simulink library "monroe_library"  (R2012b)
settings: Solver=ode45  StartTime=0.0  StopTime=10.0  RelTol=1e-3
values from neighbouring files (symbols this model uses):
  input_bit_width = ', num2str(input_bit_width))    [fft_direct_draw.m]
undefined symbols (not defined in the file or in its folder): gcbh, xlBlockLoadCallback
libraries: xbsIndex_r4 x1880, monroe_library x159, casper_library x13, xps_library x1
(part 39 of 43)

== system monroe_library/FFT_direct/direct_coeff_gen/coeff_gen_stage_3_group_2 ==
  sync : Inport
  Concat : xbsIndex_r4/Concat  num_inputs=2  dbl_ovrd=off  block_type=concat
  Concat1 : xbsIndex_r4/Concat  num_inputs=2  dbl_ovrd=off  block_type=concat
  Concat2 : xbsIndex_r4/Concat  num_inputs=2  dbl_ovrd=off  block_type=concat
  Constant : xbsIndex_r4/Constant  arith_type=Boolean  const=0  n_bits=16  bin_pt=14  explicit_period=on  period=1  equ=P=C  opselect=C  inp2=PCIN>>17  opr=+  inp1=P  carry=CIN  dbl_ovrd=off  block_type=constant
  Constant1 : xbsIndex_r4/Constant  arith_type=Boolean  const=1  n_bits=16  bin_pt=14  explicit_period=on  period=1  equ=P=C  opselect=C  inp2=PCIN>>17  opr=+  inp1=P  carry=CIN  dbl_ovrd=off  block_type=constant
  Constant3 : xbsIndex_r4/Constant  arith_type=Signed (2's comp)  const=0  n_bits=18  bin_pt=17  explicit_period=on  period=1  equ=P=C  opselect=C  inp2=PCIN>>17  opr=+  inp1=P  carry=CIN  dbl_ovrd=off  block_type=constant
  Constant4 : xbsIndex_r4/Constant  arith_type=Boolean  const=0  n_bits=16  bin_pt=14  explicit_period=on  period=1  equ=P=C  opselect=C  inp2=PCIN>>17  opr=+  inp1=P  carry=CIN  dbl_ovrd=off  block_type=constant
  Counter : xbsIndex_r4/Counter  cnt_type=Free Running  cnt_to=Inf  operation=Up  start_count=3  cnt_by_val=1  arith_type=Unsigned  n_bits=6  bin_pt=0  load_pin=off  rst=on  en=off  explicit_period=on  period=1  dbl_ovrd=off  use_behavioral_HDL=off  implementation=Fabric  block_type=counter
  Delay : xbsIndex_r4/Delay  en=off  latency=1  dbl_ovrd=off  reg_retiming=off  block_type=delay
  Dual Port RAM4 : xbsIndex_r4/Dual Port RAM  depth=128  initVector=[-1 -0.999924701839145 -0.999698818696204 -0.99932238458835 -0.998795456205172 -0.998118112900149 -0.99729045667869 -0.996312612182778 -0.995184726672197 -0.993906970002356 -0.99247953459871 -0.99090263542778 -0.989176509964781 -0.987301418157858 -0.985277642388941 -0.983105487431216 -0.98078528040323 -0.978317370719628 -0.975702130038529 -0.97293995220556 -0.970031253194544 -0.966976471044852 -0.96377606579544 -0.960430519415566 -0.956940335732209 -0.953306040354194 -0.949528180593037 -0.945607325380521 -0.941544065183021 -0.937339011912575 -0.932992798834739 -0.928506080473216 -0.923879532511287 -0.919113851690058 -0.914209755703531 -0.909167983090522 -0.903989293123443 -0.898674465693954 -0.893224301195515 -0.887639620402854 -0.881921264348355 -0.876070094195407 -0.870086991108711 -0.863972856121587 -0.857728610000272 -0.851355193105265 -0.844853565249707 -0.838224705554838 -0.831469612302545 -0.824589302785025 -0.817584813151584 -0.810457198252595 -0.803207531480645 -0.795836904608884 -0.788346427626606 -0.780737228572095 -0.773010453362737 -0.765167265622459 -0.757208846506485 -0.749136394523459 -0.740951125354959 -0.732654271672413 -0.724247082951467 -0.715730825283819 6.12323399573677e-017 -0.0122715382857198 -0.0245412285229121 -0.0368072229413589 -0.049067674327418 -0.0613207363022085 -0.0735645635996673 -0.0857973123444398 -0.0980171403295606 -0.110222207293883 -0.122410675199216 -0.134580708507126 -0.146730474455362 -0.158858143333861 -0.170961888760301 -0.183039887955141 -0.195090322016128 -0.207111376192218 -0.21910124015687 -0.231058108280671 -0.242980179903264 -0.254865659604515 -0.266712757474898 -0.278519689385053 -0.290284677254462 -0.302005949319228 -0.313681740398891 -0.325310292162263 -0.33688985339222 -0.348418680249434 -0.359895036534988 -0.371317193951837 -0.38268343236509 -0.393992040061048 -0.40524131400499 -0.416429560097637 -0.427555093430282 -0.438616238538527 -0.449611329654607 -0.46053871095824 -0.471396736825998 -0.482183772079123 -0.492898192229784 -0.503538383725717 -0.514102744193222 -0.524589682678469 -0.534997619887097 -0.545324988422046 -0.555570233019602 -0.565731810783613 -0.575808191417845 -0.585797857456439 -0.595699304492433 -0.605511041404325 -0.615231590580627 -0.624859488142386 -0.634393284163645 -0.643831542889791 -0.653172842953777 -0.662415777590172 -0.671558954847018 -0.680600997795453 -0.689540544737067 -0.698376249408973]  distributed_mem=Block RAM  init_a=0  init_b=0  rst_a=off  rst_b=off  en_a=off  en_b=off  latency=2  write_mode_A=No Read On Write  write_mode_B=No Read On Write  dbl_ovrd=off  optimize=Area  use_rpm=on  block_type=dpram
  Reinterpret : xbsIndex_r4/Reinterpret  force_arith_type=on  arith_type=Unsigned  force_bin_pt=on  bin_pt=0  block_type=reinterpret
      settings: infoedit="Changes signal type without altering the binary representation.   You can changed the signal between signed and unsigned, and relocate the binary point.<br><br>Hardware notes: In hardware this block costs nothing.<br><br>Example:  Suppose the input is 6 bits wide, signed, with 2 fractional bits, and the output is forced to unsigned with 0 fractional bits.  Then an input of -2.0 (1110.00 in binary 2's complement) becomes an output of 56 (111000 in binary)."
  Reinterpret1 : xbsIndex_r4/Reinterpret  force_arith_type=on  arith_type=Unsigned  force_bin_pt=on  bin_pt=0  block_type=reinterpret
      settings: infoedit="Changes signal type without altering the binary representation.   You can changed the signal between signed and unsigned, and relocate the binary point.<br><br>Hardware notes: In hardware this block costs nothing.<br><br>Example:  Suppose the input is 6 bits wide, signed, with 2 fractional bits, and the output is forced to unsigned with 0 fractional bits.  Then an input of -2.0 (1110.00 in binary 2's complement) becomes an output of 56 (111000 in binary)."
  count_slice : xbsIndex_r4/Slice  nbits=6  boolean_output=off  mode=Upper Bit Location + Width  bit1=0  base1=MSB of Input  bit0=0  base0=MSB of Input  dbl_ovrd=off  block_type=slice
  coeff : Outport
  wires:
  count_slice/1 -> Concat1/2, Concat/2
  Constant3/1 -> Dual Port RAM4/5, Dual Port RAM4/2
  Constant/1 -> Dual Port RAM4/6, Dual Port RAM4/3
  Reinterpret1/1 -> Concat2/2
  Dual Port RAM4/2 -> Reinterpret1/1  "xlsub2_Dual_Port_RAM4_out2"
  Reinterpret/1 -> Concat2/1
  Dual Port RAM4/1 -> Reinterpret/1  "xlsub2_Dual_Port_RAM4_out1"
  Concat1/1 -> Dual Port RAM4/4
  Concat/1 -> Dual Port RAM4/1
  Delay/1 -> coeff/1
  Concat2/1 -> Delay/1
  Constant4/1 -> Concat1/1
  Constant1/1 -> Concat/1
  Counter/1 -> count_slice/1
  sync/1 -> Counter/1

== system monroe_library/FFT_direct/direct_coeff_gen/coeff_gen_stage_3_group_3 ==
  sync : Inport
  Concat : xbsIndex_r4/Concat  num_inputs=2  dbl_ovrd=off  block_type=concat
  Concat1 : xbsIndex_r4/Concat  num_inputs=2  dbl_ovrd=off  block_type=concat
  Concat2 : xbsIndex_r4/Concat  num_inputs=2  dbl_ovrd=off  block_type=concat
  Constant : xbsIndex_r4/Constant  arith_type=Boolean  const=0  n_bits=16  bin_pt=14  explicit_period=on  period=1  equ=P=C  opselect=C  inp2=PCIN>>17  opr=+  inp1=P  carry=CIN  dbl_ovrd=off  block_type=constant
  Constant1 : xbsIndex_r4/Constant  arith_type=Boolean  const=1  n_bits=16  bin_pt=14  explicit_period=on  period=1  equ=P=C  opselect=C  inp2=PCIN>>17  opr=+  inp1=P  carry=CIN  dbl_ovrd=off  block_type=constant
  Constant3 : xbsIndex_r4/Constant  arith_type=Signed (2's comp)  const=0  n_bits=18  bin_pt=17  explicit_period=on  period=1  equ=P=C  opselect=C  inp2=PCIN>>17  opr=+  inp1=P  carry=CIN  dbl_ovrd=off  block_type=constant
  Constant4 : xbsIndex_r4/Constant  arith_type=Boolean  const=0  n_bits=16  bin_pt=14  explicit_period=on  period=1  equ=P=C  opselect=C  inp2=PCIN>>17  opr=+  inp1=P  carry=CIN  dbl_ovrd=off  block_type=constant
  Counter : xbsIndex_r4/Counter  cnt_type=Free Running  cnt_to=Inf  operation=Up  start_count=3  cnt_by_val=1  arith_type=Unsigned  n_bits=6  bin_pt=0  load_pin=off  rst=on  en=off  explicit_period=on  period=1  dbl_ovrd=off  use_behavioral_HDL=off  implementation=Fabric  block_type=counter
  Delay : xbsIndex_r4/Delay  en=off  latency=1  dbl_ovrd=off  reg_retiming=off  block_type=delay
  Dual Port RAM4 : xbsIndex_r4/Dual Port RAM  depth=128  initVector=[-0.707106781186547 -0.715730825283819 -0.724247082951467 -0.732654271672413 -0.740951125354959 -0.749136394523459 -0.757208846506485 -0.765167265622459 -0.773010453362737 -0.780737228572094 -0.788346427626606 -0.795836904608884 -0.803207531480645 -0.810457198252595 -0.817584813151584 -0.824589302785025 -0.831469612302545 -0.838224705554838 -0.844853565249707 -0.851355193105265 -0.857728610000272 -0.863972856121587 -0.870086991108711 -0.876070094195407 -0.881921264348355 -0.887639620402854 -0.893224301195515 -0.898674465693954 -0.903989293123443 -0.909167983090522 -0.914209755703531 -0.919113851690058 -0.923879532511287 -0.928506080473216 -0.932992798834739 -0.937339011912575 -0.941544065183021 -0.945607325380521 -0.949528180593037 -0.953306040354194 -0.956940335732209 -0.960430519415566 -0.96377606579544 -0.966976471044852 -0.970031253194544 -0.97293995220556 -0.975702130038529 -0.978317370719628 -0.98078528040323 -0.983105487431216 -0.985277642388941 -0.987301418157858 -0.989176509964781 -0.99090263542778 -0.99247953459871 -0.993906970002356 -0.995184726672197 -0.996312612182778 -0.99729045667869 -0.998118112900149 -0.998795456205172 -0.99932238458835 -0.999698818696204 -0.999924701839145 0.707106781186548 0.698376249408973 0.689540544737067 0.680600997795453 0.671558954847018 0.662415777590172 0.653172842953777 0.643831542889792 0.634393284163645 0.624859488142386 0.615231590580627 0.605511041404326 0.595699304492433 0.585797857456439 0.575808191417845 0.565731810783613 0.555570233019602 0.545324988422046 0.534997619887097 0.524589682678469 0.514102744193222 0.503538383725718 0.492898192229784 0.482183772079123 0.471396736825998 0.46053871095824 0.449611329654607 0.438616238538528 0.427555093430282 0.416429560097637 0.40524131400499 0.393992040061048 0.38268343236509 0.371317193951838 0.359895036534988 0.348418680249435 0.33688985339222 0.325310292162263 0.313681740398892 0.302005949319228 0.290284677254462 0.278519689385053 0.266712757474898 0.254865659604515 0.242980179903264 0.231058108280671 0.21910124015687 0.207111376192219 0.195090322016128 0.183039887955141 0.170961888760301 0.158858143333861 0.146730474455362 0.134580708507126 0.122410675199216 0.110222207293883 0.0980171403295608 0.0857973123444399 0.0735645635996675 0.0613207363022086 0.0490676743274181 0.036807222941359 0.0245412285229123 0.0122715382857199]  distributed_mem=Block RAM  init_a=0  init_b=0  rst_a=off  rst_b=off  en_a=off  en_b=off  latency=2  write_mode_A=No Read On Write  write_mode_B=No Read On Write  dbl_ovrd=off  optimize=Area  use_rpm=on  block_type=dpram
  Reinterpret : xbsIndex_r4/Reinterpret  force_arith_type=on  arith_type=Unsigned  force_bin_pt=on  bin_pt=0  block_type=reinterpret
      settings: infoedit="Changes signal type without altering the binary representation.   You can changed the signal between signed and unsigned, and relocate the binary point.<br><br>Hardware notes: In hardware this block costs nothing.<br><br>Example:  Suppose the input is 6 bits wide, signed, with 2 fractional bits, and the output is forced to unsigned with 0 fractional bits.  Then an input of -2.0 (1110.00 in binary 2's complement) becomes an output of 56 (111000 in binary)."
  Reinterpret1 : xbsIndex_r4/Reinterpret  force_arith_type=on  arith_type=Unsigned  force_bin_pt=on  bin_pt=0  block_type=reinterpret
      settings: infoedit="Changes signal type without altering the binary representation.   You can changed the signal between signed and unsigned, and relocate the binary point.<br><br>Hardware notes: In hardware this block costs nothing.<br><br>Example:  Suppose the input is 6 bits wide, signed, with 2 fractional bits, and the output is forced to unsigned with 0 fractional bits.  Then an input of -2.0 (1110.00 in binary 2's complement) becomes an output of 56 (111000 in binary)."
  count_slice : xbsIndex_r4/Slice  nbits=6  boolean_output=off  mode=Upper Bit Location + Width  bit1=0  base1=MSB of Input  bit0=0  base0=MSB of Input  dbl_ovrd=off  block_type=slice
  coeff : Outport
  wires:
  count_slice/1 -> Concat1/2, Concat/2
  Constant3/1 -> Dual Port RAM4/5, Dual Port RAM4/2
  Constant/1 -> Dual Port RAM4/6, Dual Port RAM4/3
  Reinterpret1/1 -> Concat2/2
  Dual Port RAM4/2 -> Reinterpret1/1  "xlsub2_Dual_Port_RAM4_out2"
  Reinterpret/1 -> Concat2/1
  Dual Port RAM4/1 -> Reinterpret/1  "xlsub2_Dual_Port_RAM4_out1"
  Concat1/1 -> Dual Port RAM4/4
  Concat/1 -> Dual Port RAM4/1
  Delay/1 -> coeff/1
  Concat2/1 -> Delay/1
  Constant4/1 -> Concat1/1
  Constant1/1 -> Concat/1
  Counter/1 -> count_slice/1
  sync/1 -> Counter/1

== system monroe_library/FFT_direct/direct_coeff_gen/coeff_gen_stage_3_group_4 ==
  sync : Inport
  Concat : xbsIndex_r4/Concat  num_inputs=2  dbl_ovrd=off  block_type=concat
  Concat1 : xbsIndex_r4/Concat  num_inputs=2  dbl_ovrd=off  block_type=concat
  Concat2 : xbsIndex_r4/Concat  num_inputs=2  dbl_ovrd=off  block_type=concat
  Constant : xbsIndex_r4/Constant  arith_type=Boolean  const=0  n_bits=16  bin_pt=14  explicit_period=on  period=1  equ=P=C  opselect=C  inp2=PCIN>>17  opr=+  inp1=P  carry=CIN  dbl_ovrd=off  block_type=constant
  Constant1 : xbsIndex_r4/Constant  arith_type=Boolean  const=1  n_bits=16  bin_pt=14  explicit_period=on  period=1  equ=P=C  opselect=C  inp2=PCIN>>17  opr=+  inp1=P  carry=CIN  dbl_ovrd=off  block_type=constant
  Constant3 : xbsIndex_r4/Constant  arith_type=Signed (2's comp)  const=0  n_bits=18  bin_pt=17  explicit_period=on  period=1  equ=P=C  opselect=C  inp2=PCIN>>17  opr=+  inp1=P  carry=CIN  dbl_ovrd=off  block_type=constant
  Constant4 : xbsIndex_r4/Constant  arith_type=Boolean  const=0  n_bits=16  bin_pt=14  explicit_period=on  period=1  equ=P=C  opselect=C  inp2=PCIN>>17  opr=+  inp1=P  carry=CIN  dbl_ovrd=off  block_type=constant
  Counter : xbsIndex_r4/Counter  cnt_type=Free Running  cnt_to=Inf  operation=Up  start_count=3  cnt_by_val=1  arith_type=Unsigned  n_bits=6  bin_pt=0  load_pin=off  rst=on  en=off  explicit_period=on  period=1  dbl_ovrd=off  use_behavioral_HDL=off  implementation=Fabric  block_type=counter
  Delay : xbsIndex_r4/Delay  en=off  latency=1  dbl_ovrd=off  reg_retiming=off  block_type=delay
  Dual Port RAM4 : xbsIndex_r4/Dual Port RAM  depth=128  initVector=[-0.707106781186548 -0.698376249408973 -0.689540544737067 -0.680600997795453 -0.671558954847019 -0.662415777590172 -0.653172842953777 -0.643831542889791 -0.634393284163645 -0.624859488142386 -0.615231590580627 -0.605511041404326 -0.595699304492433 -0.585797857456439 -0.575808191417845 -0.565731810783613 -0.555570233019602 -0.545324988422046 -0.534997619887097 -0.524589682678469 -0.514102744193222 -0.503538383725718 -0.492898192229784 -0.482183772079123 -0.471396736825998 -0.46053871095824 -0.449611329654607 -0.438616238538528 -0.427555093430282 -0.416429560097637 -0.40524131400499 -0.393992040061048 -0.38268343236509 -0.371317193951838 -0.359895036534988 -0.348418680249435 -0.33688985339222 -0.325310292162263 -0.313681740398891 -0.302005949319228 -0.290284677254462 -0.278519689385053 -0.266712757474898 -0.254865659604515 -0.242980179903264 -0.231058108280671 -0.21910124015687 -0.207111376192219 -0.195090322016129 -0.183039887955141 -0.170961888760301 -0.158858143333861 -0.146730474455362 -0.134580708507126 -0.122410675199216 -0.110222207293883 -0.0980171403295608 -0.0857973123444402 -0.0735645635996677 -0.0613207363022085 -0.049067674327418 -0.0368072229413588 -0.0245412285229123 -0.01227153828572 -0.707106781186547 -0.715730825283819 -0.724247082951467 -0.732654271672413 -0.740951125354959 -0.749136394523459 -0.757208846506485 -0.765167265622459 -0.773010453362737 -0.780737228572094 -0.788346427626606 -0.795836904608883 -0.803207531480645 -0.810457198252595 -0.817584813151584 -0.824589302785025 -0.831469612302545 -0.838224705554838 -0.844853565249707 -0.851355193105265 -0.857728610000272 -0.863972856121587 -0.870086991108711 -0.876070094195406 -0.881921264348355 -0.887639620402854 -0.893224301195515 -0.898674465693954 -0.903989293123443 -0.909167983090522 -0.914209755703531 -0.919113851690058 -0.923879532511287 -0.928506080473215 -0.932992798834739 -0.937339011912575 -0.941544065183021 -0.945607325380521 -0.949528180593037 -0.953306040354194 -0.956940335732209 -0.960430519415566 -0.96377606579544 -0.966976471044852 -0.970031253194544 -0.97293995220556 -0.975702130038528 -0.978317370719628 -0.98078528040323 -0.983105487431216 -0.985277642388941 -0.987301418157858 -0.989176509964781 -0.99090263542778 -0.99247953459871 -0.993906970002356 -0.995184726672197 -0.996312612182778 -0.99729045667869 -0.998118112900149 -0.998795456205172 -0.99932238458835 -0.999698818696204 -0.999924701839145]  distributed_mem=Block RAM  init_a=0  init_b=0  rst_a=off  rst_b=off  en_a=off  en_b=off  latency=2  write_mode_A=No Read On Write  write_mode_B=No Read On Write  dbl_ovrd=off  optimize=Area  use_rpm=on  block_type=dpram
  Reinterpret : xbsIndex_r4/Reinterpret  force_arith_type=on  arith_type=Unsigned  force_bin_pt=on  bin_pt=0  block_type=reinterpret
      settings: infoedit="Changes signal type without altering the binary representation.   You can changed the signal between signed and unsigned, and relocate the binary point.<br><br>Hardware notes: In hardware this block costs nothing.<br><br>Example:  Suppose the input is 6 bits wide, signed, with 2 fractional bits, and the output is forced to unsigned with 0 fractional bits.  Then an input of -2.0 (1110.00 in binary 2's complement) becomes an output of 56 (111000 in binary)."
  Reinterpret1 : xbsIndex_r4/Reinterpret  force_arith_type=on  arith_type=Unsigned  force_bin_pt=on  bin_pt=0  block_type=reinterpret
      settings: infoedit="Changes signal type without altering the binary representation.   You can changed the signal between signed and unsigned, and relocate the binary point.<br><br>Hardware notes: In hardware this block costs nothing.<br><br>Example:  Suppose the input is 6 bits wide, signed, with 2 fractional bits, and the output is forced to unsigned with 0 fractional bits.  Then an input of -2.0 (1110.00 in binary 2's complement) becomes an output of 56 (111000 in binary)."
  count_slice : xbsIndex_r4/Slice  nbits=6  boolean_output=off  mode=Upper Bit Location + Width  bit1=0  base1=MSB of Input  bit0=0  base0=MSB of Input  dbl_ovrd=off  block_type=slice
  coeff : Outport
  wires:
  count_slice/1 -> Concat1/2, Concat/2
  Constant3/1 -> Dual Port RAM4/5, Dual Port RAM4/2
  Constant/1 -> Dual Port RAM4/6, Dual Port RAM4/3
  Reinterpret1/1 -> Concat2/2
  Dual Port RAM4/2 -> Reinterpret1/1  "xlsub2_Dual_Port_RAM4_out2"
  Reinterpret/1 -> Concat2/1
  Dual Port RAM4/1 -> Reinterpret/1  "xlsub2_Dual_Port_RAM4_out1"
  Concat1/1 -> Dual Port RAM4/4
  Concat/1 -> Dual Port RAM4/1
  Delay/1 -> coeff/1
  Concat2/1 -> Delay/1
  Constant4/1 -> Concat1/1
  Constant1/1 -> Concat/1
  Counter/1 -> count_slice/1
  sync/1 -> Counter/1

== system monroe_library/FFT_direct/stage_1/uncram_coeff ==
  in : Inport
  signal1 : xbsIndex_r4/Slice  nbits=36  boolean_output=off  mode=Upper Bit Location + Width  bit1=-0  base1=MSB of Input  bit0=-0  base0=MSB of Input  dbl_ovrd=off  block_type=slice
  signal2 : xbsIndex_r4/Slice  nbits=36  boolean_output=off  mode=Upper Bit Location + Width  bit1=-36  base1=MSB of Input  bit0=-36  base0=MSB of Input  dbl_ovrd=off  block_type=slice
  signal3 : xbsIndex_r4/Slice  nbits=36  boolean_output=off  mode=Upper Bit Location + Width  bit1=-72  base1=MSB of Input  bit0=-72  base0=MSB of Input  dbl_ovrd=off  block_type=slice
  signal4 : xbsIndex_r4/Slice  nbits=36  boolean_output=off  mode=Upper Bit Location + Width  bit1=-108  base1=MSB of Input  bit0=-108  base0=MSB of Input  dbl_ovrd=off  block_type=slice
  out0 : Outport
  out1 : Outport  Port=2
  out2 : Outport  Port=3
  out3 : Outport  Port=4
  wires:
  in/1 -> signal4/1, signal3/1, signal2/1, signal1/1
  signal4/1 -> out3/1
  signal3/1 -> out2/1
  signal2/1 -> out1/1
  signal1/1 -> out0/1

== system monroe_library/FFT_direct/stage_2/uncram_coeff ==
  in : Inport
  signal1 : xbsIndex_r4/Slice  nbits=36  boolean_output=off  mode=Upper Bit Location + Width  bit1=-0  base1=MSB of Input  bit0=-0  base0=MSB of Input  dbl_ovrd=off  block_type=slice
  signal2 : xbsIndex_r4/Slice  nbits=36  boolean_output=off  mode=Upper Bit Location + Width  bit1=-36  base1=MSB of Input  bit0=-36  base0=MSB of Input  dbl_ovrd=off  block_type=slice
  signal3 : xbsIndex_r4/Slice  nbits=36  boolean_output=off  mode=Upper Bit Location + Width  bit1=-72  base1=MSB of Input  bit0=-72  base0=MSB of Input  dbl_ovrd=off  block_type=slice
  signal4 : xbsIndex_r4/Slice  nbits=36  boolean_output=off  mode=Upper Bit Location + Width  bit1=-108  base1=MSB of Input  bit0=-108  base0=MSB of Input  dbl_ovrd=off  block_type=slice
  out0 : Outport
  out1 : Outport  Port=2
  out2 : Outport  Port=3
  out3 : Outport  Port=4
  wires:
  in/1 -> signal4/1, signal3/1, signal2/1, signal1/1
  signal4/1 -> out3/1
  signal3/1 -> out2/1
  signal2/1 -> out1/1
  signal1/1 -> out0/1

== system monroe_library/FFT_direct/stage_3/uncram_coeff ==
  in : Inport
  signal1 : xbsIndex_r4/Slice  nbits=36  boolean_output=off  mode=Upper Bit Location + Width  bit1=-0  base1=MSB of Input  bit0=-0  base0=MSB of Input  dbl_ovrd=off  block_type=slice
  signal2 : xbsIndex_r4/Slice  nbits=36  boolean_output=off  mode=Upper Bit Location + Width  bit1=-36  base1=MSB of Input  bit0=-36  base0=MSB of Input  dbl_ovrd=off  block_type=slice
  signal3 : xbsIndex_r4/Slice  nbits=36  boolean_output=off  mode=Upper Bit Location + Width  bit1=-72  base1=MSB of Input  bit0=-72  base0=MSB of Input  dbl_ovrd=off  block_type=slice
  signal4 : xbsIndex_r4/Slice  nbits=36  boolean_output=off  mode=Upper Bit Location + Width  bit1=-108  base1=MSB of Input  bit0=-108  base0=MSB of Input  dbl_ovrd=off  block_type=slice
  out0 : Outport
  out1 : Outport  Port=2
  out2 : Outport  Port=3
  out3 : Outport  Port=4
  wires:
  in/1 -> signal4/1, signal3/1, signal2/1, signal1/1
  signal4/1 -> out3/1
  signal3/1 -> out2/1
  signal2/1 -> out1/1
  signal1/1 -> out0/1

== system monroe_library/biplex_4x_unscr/dual_bit_reverse/bit_reverse_1 ==
  in : Inport
  concat : xbsIndex_r4/Concat  num_inputs=8  dbl_ovrd=off  block_type=concat
  slice1 : xbsIndex_r4/Slice  nbits=1  boolean_output=on  mode=Upper Bit Location + Width  bit1=-0  base1=MSB of Input  bit0=-0  base0=MSB of Input  dbl_ovrd=off  block_type=slice
  slice2 : xbsIndex_r4/Slice  nbits=1  boolean_output=on  mode=Upper Bit Location + Width  bit1=-1  base1=MSB of Input  bit0=-1  base0=MSB of Input  dbl_ovrd=off  block_type=slice
  slice3 : xbsIndex_r4/Slice  nbits=1  boolean_output=on  mode=Upper Bit Location + Width  bit1=-2  base1=MSB of Input  bit0=-2  base0=MSB of Input  dbl_ovrd=off  block_type=slice
  slice4 : xbsIndex_r4/Slice  nbits=1  boolean_output=on  mode=Upper Bit Location + Width  bit1=-3  base1=MSB of Input  bit0=-3  base0=MSB of Input  dbl_ovrd=off  block_type=slice
  slice5 : xbsIndex_r4/Slice  nbits=1  boolean_output=on  mode=Upper Bit Location + Width  bit1=-4  base1=MSB of Input  bit0=-4  base0=MSB of Input  dbl_ovrd=off  block_type=slice
  slice6 : xbsIndex_r4/Slice  nbits=1  boolean_output=on  mode=Upper Bit Location + Width  bit1=-5  base1=MSB of Input  bit0=-5  base0=MSB of Input  dbl_ovrd=off  block_type=slice
  slice7 : xbsIndex_r4/Slice  nbits=1  boolean_output=on  mode=Upper Bit Location + Width  bit1=-6  base1=MSB of Input  bit0=-6  base0=MSB of Input  dbl_ovrd=off  block_type=slice
  slice8 : xbsIndex_r4/Slice  nbits=1  boolean_output=on  mode=Upper Bit Location + Width  bit1=-7  base1=MSB of Input  bit0=-7  base0=MSB of Input  dbl_ovrd=off  block_type=slice
  out : Outport
  wires:
  in/1 -> slice8/1, slice7/1, slice6/1, slice5/1, slice4/1, slice3/1, slice2/1, slice1/1
  concat/1 -> out/1
  slice1/1 -> concat/8
  slice2/1 -> concat/7
  slice3/1 -> concat/6
  slice4/1 -> concat/5
  slice5/1 -> concat/4
  slice6/1 -> concat/3
  slice7/1 -> concat/2
  slice8/1 -> concat/1

== system monroe_library/biplex_4x_unscr/dual_bit_reverse/bit_reverse_2 ==
  in : Inport
  concat : xbsIndex_r4/Concat  num_inputs=8  dbl_ovrd=off  block_type=concat
  slice1 : xbsIndex_r4/Slice  nbits=1  boolean_output=on  mode=Upper Bit Location + Width  bit1=-0  base1=MSB of Input  bit0=-0  base0=MSB of Input  dbl_ovrd=off  block_type=slice
  slice2 : xbsIndex_r4/Slice  nbits=1  boolean_output=on  mode=Upper Bit Location + Width  bit1=-1  base1=MSB of Input  bit0=-1  base0=MSB of Input  dbl_ovrd=off  block_type=slice
  slice3 : xbsIndex_r4/Slice  nbits=1  boolean_output=on  mode=Upper Bit Location + Width  bit1=-2  base1=MSB of Input  bit0=-2  base0=MSB of Input  dbl_ovrd=off  block_type=slice
  slice4 : xbsIndex_r4/Slice  nbits=1  boolean_output=on  mode=Upper Bit Location + Width  bit1=-3  base1=MSB of Input  bit0=-3  base0=MSB of Input  dbl_ovrd=off  block_type=slice
  slice5 : xbsIndex_r4/Slice  nbits=1  boolean_output=on  mode=Upper Bit Location + Width  bit1=-4  base1=MSB of Input  bit0=-4  base0=MSB of Input  dbl_ovrd=off  block_type=slice
  slice6 : xbsIndex_r4/Slice  nbits=1  boolean_output=on  mode=Upper Bit Location + Width  bit1=-5  base1=MSB of Input  bit0=-5  base0=MSB of Input  dbl_ovrd=off  block_type=slice
  slice7 : xbsIndex_r4/Slice  nbits=1  boolean_output=on  mode=Upper Bit Location + Width  bit1=-6  base1=MSB of Input  bit0=-6  base0=MSB of Input  dbl_ovrd=off  block_type=slice
  slice8 : xbsIndex_r4/Slice  nbits=1  boolean_output=on  mode=Upper Bit Location + Width  bit1=-7  base1=MSB of Input  bit0=-7  base0=MSB of Input  dbl_ovrd=off  block_type=slice
  out : Outport
  wires:
  in/1 -> slice8/1, slice7/1, slice6/1, slice5/1, slice4/1, slice3/1, slice2/1, slice1/1
  concat/1 -> out/1
  slice1/1 -> concat/8
  slice2/1 -> concat/7
  slice3/1 -> concat/6
  slice4/1 -> concat/5
  slice5/1 -> concat/4
  slice6/1 -> concat/3
  slice7/1 -> concat/2
  slice8/1 -> concat/1

== system monroe_library/pfb_fir_real/coeff_gen_0_15/cram_lower ==
  in0 : Inport
  in1 : Inport  Port=2
  in2 : Inport  Port=3
  in3 : Inport  Port=4
  concat : xbsIndex_r4/Concat  num_inputs=4  dbl_ovrd=off  block_type=concat
  reinterpret_{1..4} (4 alike) : xbsIndex_r4/Reinterpret  force_arith_type=on  arith_type=Unsigned  force_bin_pt=on  bin_pt=0  block_type=reinterpret
      settings: infoedit="Changes signal type without altering the binary representation.   You can changed the signal between signed and unsigned, and relocate the binary point.<br><br>Hardware notes: In hardware this block costs nothing.<br><br>Example:  Suppose the input is 6 bits wide, signed, with 2 fractional bits, and the output is forced to unsigned with 0 fractional bits.  Then an input of -2.0 (1110.00 in binary 2's complement) becomes an output of 56 (111000 in binary)."
  out : Outport
  wires:
  concat/1 -> out/1
  reinterpret_4/1 -> concat/4
  reinterpret_3/1 -> concat/3
  reinterpret_2/1 -> concat/2
  reinterpret_1/1 -> concat/1
  in3/1 -> reinterpret_4/1
  in2/1 -> reinterpret_3/1
  in1/1 -> reinterpret_2/1
  in0/1 -> reinterpret_1/1

== system monroe_library/pfb_fir_real/coeff_gen_0_15/cram_upper ==
  in0 : Inport
  in1 : Inport  Port=2
  in2 : Inport  Port=3
  in3 : Inport  Port=4
  concat : xbsIndex_r4/Concat  num_inputs=4  dbl_ovrd=off  block_type=concat
  reinterpret_{1..4} (4 alike) : xbsIndex_r4/Reinterpret  force_arith_type=on  arith_type=Unsigned  force_bin_pt=on  bin_pt=0  block_type=reinterpret
      settings: infoedit="Changes signal type without altering the binary representation.   You can changed the signal between signed and unsigned, and relocate the binary point.<br><br>Hardware notes: In hardware this block costs nothing.<br><br>Example:  Suppose the input is 6 bits wide, signed, with 2 fractional bits, and the output is forced to unsigned with 0 fractional bits.  Then an input of -2.0 (1110.00 in binary 2's complement) becomes an output of 56 (111000 in binary)."
  out : Outport
  wires:
  concat/1 -> out/1
  reinterpret_4/1 -> concat/4
  reinterpret_3/1 -> concat/3
  reinterpret_2/1 -> concat/2
  reinterpret_1/1 -> concat/1
  in3/1 -> reinterpret_4/1
  in2/1 -> reinterpret_3/1
  in1/1 -> reinterpret_2/1
  in0/1 -> reinterpret_1/1

== system monroe_library/pfb_fir_real/coeff_gen_1_14/cram_lower ==
  in0 : Inport
  in1 : Inport  Port=2
  in2 : Inport  Port=3
  in3 : Inport  Port=4
  concat : xbsIndex_r4/Concat  num_inputs=4  dbl_ovrd=off  block_type=concat
  reinterpret_{1..4} (4 alike) : xbsIndex_r4/Reinterpret  force_arith_type=on  arith_type=Unsigned  force_bin_pt=on  bin_pt=0  block_type=reinterpret
      settings: infoedit="Changes signal type without altering the binary representation.   You can changed the signal between signed and unsigned, and relocate the binary point.<br><br>Hardware notes: In hardware this block costs nothing.<br><br>Example:  Suppose the input is 6 bits wide, signed, with 2 fractional bits, and the output is forced to unsigned with 0 fractional bits.  Then an input of -2.0 (1110.00 in binary 2's complement) becomes an output of 56 (111000 in binary)."
  out : Outport
  wires:
  concat/1 -> out/1
  reinterpret_4/1 -> concat/4
  reinterpret_3/1 -> concat/3
  reinterpret_2/1 -> concat/2
  reinterpret_1/1 -> concat/1
  in3/1 -> reinterpret_4/1
  in2/1 -> reinterpret_3/1
  in1/1 -> reinterpret_2/1
  in0/1 -> reinterpret_1/1

== system monroe_library/pfb_fir_real/coeff_gen_1_14/cram_upper ==
  in0 : Inport
  in1 : Inport  Port=2
  in2 : Inport  Port=3
  in3 : Inport  Port=4
  concat : xbsIndex_r4/Concat  num_inputs=4  dbl_ovrd=off  block_type=concat
  reinterpret_{1..4} (4 alike) : xbsIndex_r4/Reinterpret  force_arith_type=on  arith_type=Unsigned  force_bin_pt=on  bin_pt=0  block_type=reinterpret
      settings: infoedit="Changes signal type without altering the binary representation.   You can changed the signal between signed and unsigned, and relocate the binary point.<br><br>Hardware notes: In hardware this block costs nothing.<br><br>Example:  Suppose the input is 6 bits wide, signed, with 2 fractional bits, and the output is forced to unsigned with 0 fractional bits.  Then an input of -2.0 (1110.00 in binary 2's complement) becomes an output of 56 (111000 in binary)."
  out : Outport
  wires:
  concat/1 -> out/1
  reinterpret_4/1 -> concat/4
  reinterpret_3/1 -> concat/3
  reinterpret_2/1 -> concat/2
  reinterpret_1/1 -> concat/1
  in3/1 -> reinterpret_4/1
  in2/1 -> reinterpret_3/1
  in1/1 -> reinterpret_2/1
  in0/1 -> reinterpret_1/1

== system monroe_library/pfb_fir_real/coeff_gen_2_13/cram_lower ==
  in0 : Inport
  in1 : Inport  Port=2
  in2 : Inport  Port=3
  in3 : Inport  Port=4
  concat : xbsIndex_r4/Concat  num_inputs=4  dbl_ovrd=off  block_type=concat
  reinterpret_{1..4} (4 alike) : xbsIndex_r4/Reinterpret  force_arith_type=on  arith_type=Unsigned  force_bin_pt=on  bin_pt=0  block_type=reinterpret
      settings: infoedit="Changes signal type without altering the binary representation.   You can changed the signal between signed and unsigned, and relocate the binary point.<br><br>Hardware notes: In hardware this block costs nothing.<br><br>Example:  Suppose the input is 6 bits wide, signed, with 2 fractional bits, and the output is forced to unsigned with 0 fractional bits.  Then an input of -2.0 (1110.00 in binary 2's complement) becomes an output of 56 (111000 in binary)."
  out : Outport
  wires:
  concat/1 -> out/1
  reinterpret_4/1 -> concat/4
  reinterpret_3/1 -> concat/3
  reinterpret_2/1 -> concat/2
  reinterpret_1/1 -> concat/1
  in3/1 -> reinterpret_4/1
  in2/1 -> reinterpret_3/1
  in1/1 -> reinterpret_2/1
  in0/1 -> reinterpret_1/1

== system monroe_library/pfb_fir_real/coeff_gen_2_13/cram_upper ==
  in0 : Inport
  in1 : Inport  Port=2
  in2 : Inport  Port=3
  in3 : Inport  Port=4
  concat : xbsIndex_r4/Concat  num_inputs=4  dbl_ovrd=off  block_type=concat
  reinterpret_{1..4} (4 alike) : xbsIndex_r4/Reinterpret  force_arith_type=on  arith_type=Unsigned  force_bin_pt=on  bin_pt=0  block_type=reinterpret
      settings: infoedit="Changes signal type without altering the binary representation.   You can changed the signal between signed and unsigned, and relocate the binary point.<br><br>Hardware notes: In hardware this block costs nothing.<br><br>Example:  Suppose the input is 6 bits wide, signed, with 2 fractional bits, and the output is forced to unsigned with 0 fractional bits.  Then an input of -2.0 (1110.00 in binary 2's complement) becomes an output of 56 (111000 in binary)."
  out : Outport
  wires:
  concat/1 -> out/1
  reinterpret_4/1 -> concat/4
  reinterpret_3/1 -> concat/3
  reinterpret_2/1 -> concat/2
  reinterpret_1/1 -> concat/1
  in3/1 -> reinterpret_4/1
  in2/1 -> reinterpret_3/1
  in1/1 -> reinterpret_2/1
  in0/1 -> reinterpret_1/1

== system monroe_library/pfb_fir_real/coeff_gen_3_12/cram_lower ==
  in0 : Inport
  in1 : Inport  Port=2
  in2 : Inport  Port=3
  in3 : Inport  Port=4
  concat : xbsIndex_r4/Concat  num_inputs=4  dbl_ovrd=off  block_type=concat
  reinterpret_{1..4} (4 alike) : xbsIndex_r4/Reinterpret  force_arith_type=on  arith_type=Unsigned  force_bin_pt=on  bin_pt=0  block_type=reinterpret
      settings: infoedit="Changes signal type without altering the binary representation.   You can changed the signal between signed and unsigned, and relocate the binary point.<br><br>Hardware notes: In hardware this block costs nothing.<br><br>Example:  Suppose the input is 6 bits wide, signed, with 2 fractional bits, and the output is forced to unsigned with 0 fractional bits.  Then an input of -2.0 (1110.00 in binary 2's complement) becomes an output of 56 (111000 in binary)."
  out : Outport
  wires:
  concat/1 -> out/1
  reinterpret_4/1 -> concat/4
  reinterpret_3/1 -> concat/3
  reinterpret_2/1 -> concat/2
  reinterpret_1/1 -> concat/1
  in3/1 -> reinterpret_4/1
  in2/1 -> reinterpret_3/1
  in1/1 -> reinterpret_2/1
  in0/1 -> reinterpret_1/1

== system monroe_library/pfb_fir_real/coeff_gen_3_12/cram_upper ==
  in0 : Inport
  in1 : Inport  Port=2
  in2 : Inport  Port=3
  in3 : Inport  Port=4
  concat : xbsIndex_r4/Concat  num_inputs=4  dbl_ovrd=off  block_type=concat
  reinterpret_{1..4} (4 alike) : xbsIndex_r4/Reinterpret  force_arith_type=on  arith_type=Unsigned  force_bin_pt=on  bin_pt=0  block_type=reinterpret
      settings: infoedit="Changes signal type without altering the binary representation.   You can changed the signal between signed and unsigned, and relocate the binary point.<br><br>Hardware notes: In hardware this block costs nothing.<br><br>Example:  Suppose the input is 6 bits wide, signed, with 2 fractional bits, and the output is forced to unsigned with 0 fractional bits.  Then an input of -2.0 (1110.00 in binary 2's complement) becomes an output of 56 (111000 in binary)."
  out : Outport
  wires:
  concat/1 -> out/1
  reinterpret_4/1 -> concat/4
  reinterpret_3/1 -> concat/3
  reinterpret_2/1 -> concat/2
  reinterpret_1/1 -> concat/1
  in3/1 -> reinterpret_4/1
  in2/1 -> reinterpret_3/1
  in1/1 -> reinterpret_2/1
  in0/1 -> reinterpret_1/1

== system monroe_library/pfb_fir_real/coeff_gen_4_11/cram_lower ==
  in0 : Inport
  in1 : Inport  Port=2
  in2 : Inport  Port=3
  in3 : Inport  Port=4
  concat : xbsIndex_r4/Concat  num_inputs=4  dbl_ovrd=off  block_type=concat
  reinterpret_{1..4} (4 alike) : xbsIndex_r4/Reinterpret  force_arith_type=on  arith_type=Unsigned  force_bin_pt=on  bin_pt=0  block_type=reinterpret
      settings: infoedit="Changes signal type without altering the binary representation.   You can changed the signal between signed and unsigned, and relocate the binary point.<br><br>Hardware notes: In hardware this block costs nothing.<br><br>Example:  Suppose the input is 6 bits wide, signed, with 2 fractional bits, and the output is forced to unsigned with 0 fractional bits.  Then an input of -2.0 (1110.00 in binary 2's complement) becomes an output of 56 (111000 in binary)."
  out : Outport
  wires:
  concat/1 -> out/1
  reinterpret_4/1 -> concat/4
  reinterpret_3/1 -> concat/3
  reinterpret_2/1 -> concat/2
  reinterpret_1/1 -> concat/1
  in3/1 -> reinterpret_4/1
  in2/1 -> reinterpret_3/1
  in1/1 -> reinterpret_2/1
  in0/1 -> reinterpret_1/1

== system monroe_library/pfb_fir_real/coeff_gen_4_11/cram_upper ==
  in0 : Inport
  in1 : Inport  Port=2
  in2 : Inport  Port=3
  in3 : Inport  Port=4
  concat : xbsIndex_r4/Concat  num_inputs=4  dbl_ovrd=off  block_type=concat
  reinterpret_{1..4} (4 alike) : xbsIndex_r4/Reinterpret  force_arith_type=on  arith_type=Unsigned  force_bin_pt=on  bin_pt=0  block_type=reinterpret
      settings: infoedit="Changes signal type without altering the binary representation.   You can changed the signal between signed and unsigned, and relocate the binary point.<br><br>Hardware notes: In hardware this block costs nothing.<br><br>Example:  Suppose the input is 6 bits wide, signed, with 2 fractional bits, and the output is forced to unsigned with 0 fractional bits.  Then an input of -2.0 (1110.00 in binary 2's complement) becomes an output of 56 (111000 in binary)."
  out : Outport
  wires:
  concat/1 -> out/1
  reinterpret_4/1 -> concat/4
  reinterpret_3/1 -> concat/3
  reinterpret_2/1 -> concat/2
  reinterpret_1/1 -> concat/1
  in3/1 -> reinterpret_4/1
  in2/1 -> reinterpret_3/1
  in1/1 -> reinterpret_2/1
  in0/1 -> reinterpret_1/1

== system monroe_library/pfb_fir_real/coeff_gen_5_10/cram_lower ==
  in0 : Inport
  in1 : Inport  Port=2
  in2 : Inport  Port=3
  in3 : Inport  Port=4
  concat : xbsIndex_r4/Concat  num_inputs=4  dbl_ovrd=off  block_type=concat
  reinterpret_{1..4} (4 alike) : xbsIndex_r4/Reinterpret  force_arith_type=on  arith_type=Unsigned  force_bin_pt=on  bin_pt=0  block_type=reinterpret
      settings: infoedit="Changes signal type without altering the binary representation.   You can changed the signal between signed and unsigned, and relocate the binary point.<br><br>Hardware notes: In hardware this block costs nothing.<br><br>Example:  Suppose the input is 6 bits wide, signed, with 2 fractional bits, and the output is forced to unsigned with 0 fractional bits.  Then an input of -2.0 (1110.00 in binary 2's complement) becomes an output of 56 (111000 in binary)."
  out : Outport
  wires:
  concat/1 -> out/1
  reinterpret_4/1 -> concat/4
  reinterpret_3/1 -> concat/3
  reinterpret_2/1 -> concat/2
  reinterpret_1/1 -> concat/1
  in3/1 -> reinterpret_4/1
  in2/1 -> reinterpret_3/1
  in1/1 -> reinterpret_2/1
  in0/1 -> reinterpret_1/1

== system monroe_library/pfb_fir_real/coeff_gen_5_10/cram_upper ==
  in0 : Inport
  in1 : Inport  Port=2
  in2 : Inport  Port=3
  in3 : Inport  Port=4
  concat : xbsIndex_r4/Concat  num_inputs=4  dbl_ovrd=off  block_type=concat
  reinterpret_{1..4} (4 alike) : xbsIndex_r4/Reinterpret  force_arith_type=on  arith_type=Unsigned  force_bin_pt=on  bin_pt=0  block_type=reinterpret
      settings: infoedit="Changes signal type without altering the binary representation.   You can changed the signal between signed and unsigned, and relocate the binary point.<br><br>Hardware notes: In hardware this block costs nothing.<br><br>Example:  Suppose the input is 6 bits wide, signed, with 2 fractional bits, and the output is forced to unsigned with 0 fractional bits.  Then an input of -2.0 (1110.00 in binary 2's complement) becomes an output of 56 (111000 in binary)."
  out : Outport
  wires:
  concat/1 -> out/1
  reinterpret_4/1 -> concat/4
  reinterpret_3/1 -> concat/3
  reinterpret_2/1 -> concat/2
  reinterpret_1/1 -> concat/1
  in3/1 -> reinterpret_4/1
  in2/1 -> reinterpret_3/1
  in1/1 -> reinterpret_2/1
  in0/1 -> reinterpret_1/1

== system monroe_library/pfb_fir_real/coeff_gen_6_9/cram_lower ==
  in0 : Inport
  in1 : Inport  Port=2
  in2 : Inport  Port=3
  in3 : Inport  Port=4
  concat : xbsIndex_r4/Concat  num_inputs=4  dbl_ovrd=off  block_type=concat
  reinterpret_{1..4} (4 alike) : xbsIndex_r4/Reinterpret  force_arith_type=on  arith_type=Unsigned  force_bin_pt=on  bin_pt=0  block_type=reinterpret
      settings: infoedit="Changes signal type without altering the binary representation.   You can changed the signal between signed and unsigned, and relocate the binary point.<br><br>Hardware notes: In hardware this block costs nothing.<br><br>Example:  Suppose the input is 6 bits wide, signed, with 2 fractional bits, and the output is forced to unsigned with 0 fractional bits.  Then an input of -2.0 (1110.00 in binary 2's complement) becomes an output of 56 (111000 in binary)."
  out : Outport
  wires:
  concat/1 -> out/1
  reinterpret_4/1 -> concat/4
  reinterpret_3/1 -> concat/3
  reinterpret_2/1 -> concat/2
  reinterpret_1/1 -> concat/1
  in3/1 -> reinterpret_4/1
  in2/1 -> reinterpret_3/1
  in1/1 -> reinterpret_2/1
  in0/1 -> reinterpret_1/1

== system monroe_library/pfb_fir_real/coeff_gen_6_9/cram_upper ==
  in0 : Inport
  in1 : Inport  Port=2
  in2 : Inport  Port=3
  in3 : Inport  Port=4
  concat : xbsIndex_r4/Concat  num_inputs=4  dbl_ovrd=off  block_type=concat
  reinterpret_{1..4} (4 alike) : xbsIndex_r4/Reinterpret  force_arith_type=on  arith_type=Unsigned  force_bin_pt=on  bin_pt=0  block_type=reinterpret
      settings: infoedit="Changes signal type without altering the binary representation.   You can changed the signal between signed and unsigned, and relocate the binary point.<br><br>Hardware notes: In hardware this block costs nothing.<br><br>Example:  Suppose the input is 6 bits wide, signed, with 2 fractional bits, and the output is forced to unsigned with 0 fractional bits.  Then an input of -2.0 (1110.00 in binary 2's complement) becomes an output of 56 (111000 in binary)."
  out : Outport
  wires:
  concat/1 -> out/1
  reinterpret_4/1 -> concat/4
  reinterpret_3/1 -> concat/3
  reinterpret_2/1 -> concat/2
  reinterpret_1/1 -> concat/1
  in3/1 -> reinterpret_4/1
  in2/1 -> reinterpret_3/1
  in1/1 -> reinterpret_2/1
  in0/1 -> reinterpret_1/1

== system monroe_library/pfb_fir_real/coeff_gen_7_8/cram_lower ==
  in0 : Inport
  in1 : Inport  Port=2
  in2 : Inport  Port=3
  in3 : Inport  Port=4
  concat : xbsIndex_r4/Concat  num_inputs=4  dbl_ovrd=off  block_type=concat
  reinterpret_{1..4} (4 alike) : xbsIndex_r4/Reinterpret  force_arith_type=on  arith_type=Unsigned  force_bin_pt=on  bin_pt=0  block_type=reinterpret
      settings: infoedit="Changes signal type without altering the binary representation.   You can changed the signal between signed and unsigned, and relocate the binary point.<br><br>Hardware notes: In hardware this block costs nothing.<br><br>Example:  Suppose the input is 6 bits wide, signed, with 2 fractional bits, and the output is forced to unsigned with 0 fractional bits.  Then an input of -2.0 (1110.00 in binary 2's complement) becomes an output of 56 (111000 in binary)."
  out : Outport
  wires:
  concat/1 -> out/1
  reinterpret_4/1 -> concat/4
  reinterpret_3/1 -> concat/3
  reinterpret_2/1 -> concat/2
  reinterpret_1/1 -> concat/1
  in3/1 -> reinterpret_4/1
  in2/1 -> reinterpret_3/1
  in1/1 -> reinterpret_2/1
  in0/1 -> reinterpret_1/1

== system monroe_library/pfb_fir_real/coeff_gen_7_8/cram_upper ==
  in0 : Inport
  in1 : Inport  Port=2
  in2 : Inport  Port=3
  in3 : Inport  Port=4
  concat : xbsIndex_r4/Concat  num_inputs=4  dbl_ovrd=off  block_type=concat
  reinterpret_{1..4} (4 alike) : xbsIndex_r4/Reinterpret  force_arith_type=on  arith_type=Unsigned  force_bin_pt=on  bin_pt=0  block_type=reinterpret
      settings: infoedit="Changes signal type without altering the binary representation.   You can changed the signal between signed and unsigned, and relocate the binary point.<br><br>Hardware notes: In hardware this block costs nothing.<br><br>Example:  Suppose the input is 6 bits wide, signed, with 2 fractional bits, and the output is forced to unsigned with 0 fractional bits.  Then an input of -2.0 (1110.00 in binary 2's complement) becomes an output of 56 (111000 in binary)."
  out : Outport
  wires:
  concat/1 -> out/1
  reinterpret_4/1 -> concat/4
  reinterpret_3/1 -> concat/3
  reinterpret_2/1 -> concat/2
  reinterpret_1/1 -> concat/1
  in3/1 -> reinterpret_4/1
  in2/1 -> reinterpret_3/1
  in1/1 -> reinterpret_2/1
  in0/1 -> reinterpret_1/1

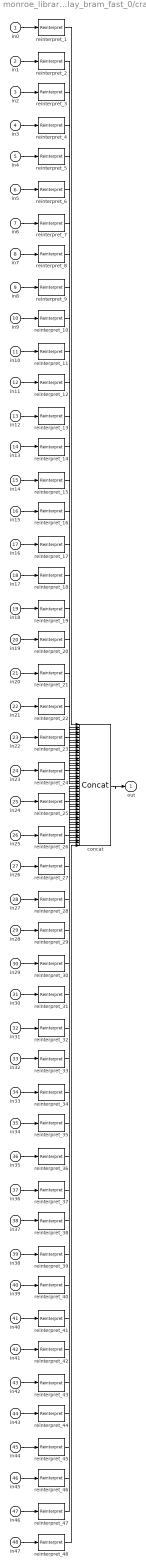
== system monroe_library/pfb_fir_real/multi_delay_bram_fast_0/cram ==
  in0 : Inport
  in1 : Inport  Port=2
  in2 : Inport  Port=3
  in3 : Inport  Port=4
  in4 : Inport  Port=5
  in5 : Inport  Port=6
  in6 : Inport  Port=7
  in7 : Inport  Port=8
  in8 : Inport  Port=9
  in9 : Inport  Port=10
  in10 : Inport  Port=11
  in11 : Inport  Port=12
  in12 : Inport  Port=13
  in13 : Inport  Port=14
  in14 : Inport  Port=15
  in15 : Inport  Port=16
  in16 : Inport  Port=17
  in17 : Inport  Port=18
  in18 : Inport  Port=19
  in19 : Inport  Port=20
  in20 : Inport  Port=21
  in21 : Inport  Port=22
  in22 : Inport  Port=23
  in23 : Inport  Port=24
  in24 : Inport  Port=25
  in25 : Inport  Port=26
  in26 : Inport  Port=27
  in27 : Inport  Port=28
  in28 : Inport  Port=29
  in29 : Inport  Port=30
  in30 : Inport  Port=31
  in31 : Inport  Port=32
  in32 : Inport  Port=33
  in33 : Inport  Port=34
  in34 : Inport  Port=35
  in35 : Inport  Port=36
  in36 : Inport  Port=37
  in37 : Inport  Port=38
  in38 : Inport  Port=39
  in39 : Inport  Port=40
  in40 : Inport  Port=41
  in41 : Inport  Port=42
  in42 : Inport  Port=43
  in43 : Inport  Port=44
  in44 : Inport  Port=45
  in45 : Inport  Port=46
  in46 : Inport  Port=47
  in47 : Inport  Port=48
  concat : xbsIndex_r4/Concat  num_inputs=48  dbl_ovrd=off  block_type=concat
  reinterpret_{1..48} (48 alike) : xbsIndex_r4/Reinterpret  force_arith_type=on  arith_type=Unsigned  force_bin_pt=on  bin_pt=0  block_type=reinterpret
      settings: infoedit="Changes signal type without altering the binary representation.   You can changed the signal between signed and unsigned, and relocate the binary point.<br><br>Hardware notes: In hardware this block costs nothing.<br><br>Example:  Suppose the input is 6 bits wide, signed, with 2 fractional bits, and the output is forced to unsigned with 0 fractional bits.  Then an input of -2.0 (1110.00 in binary 2's complement) becomes an output of 56 (111000 in binary)."
  out : Outport
  wires:
  concat/1 -> out/1
  reinterpret_48/1 -> concat/48
  reinterpret_47/1 -> concat/47
  reinterpret_46/1 -> concat/46
  reinterpret_45/1 -> concat/45
  reinterpret_44/1 -> concat/44
  reinterpret_43/1 -> concat/43
  reinterpret_42/1 -> concat/42
  reinterpret_41/1 -> concat/41
  reinterpret_40/1 -> concat/40
  reinterpret_39/1 -> concat/39
  reinterpret_38/1 -> concat/38
  reinterpret_37/1 -> concat/37
  reinterpret_36/1 -> concat/36
  reinterpret_35/1 -> concat/35
  reinterpret_34/1 -> concat/34
  reinterpret_33/1 -> concat/33
  reinterpret_32/1 -> concat/32
  reinterpret_31/1 -> concat/31
  reinterpret_30/1 -> concat/30
  reinterpret_29/1 -> concat/29
  reinterpret_28/1 -> concat/28
  reinterpret_27/1 -> concat/27
  reinterpret_26/1 -> concat/26
  reinterpret_25/1 -> concat/25
  reinterpret_24/1 -> concat/24
  reinterpret_23/1 -> concat/23
  reinterpret_22/1 -> concat/22
  reinterpret_21/1 -> concat/21
  reinterpret_20/1 -> concat/20
  reinterpret_19/1 -> concat/19
  reinterpret_18/1 -> concat/18
  reinterpret_17/1 -> concat/17
  reinterpret_16/1 -> concat/16
  reinterpret_15/1 -> concat/15
  reinterpret_14/1 -> concat/14
  reinterpret_13/1 -> concat/13
  reinterpret_12/1 -> concat/12
  reinterpret_11/1 -> concat/11
  reinterpret_10/1 -> concat/10
  reinterpret_9/1 -> concat/9
  reinterpret_8/1 -> concat/8
  reinterpret_7/1 -> concat/7
  reinterpret_6/1 -> concat/6
  reinterpret_5/1 -> concat/5
  reinterpret_4/1 -> concat/4
  reinterpret_3/1 -> concat/3
  reinterpret_2/1 -> concat/2
  reinterpret_1/1 -> concat/1
  in47/1 -> reinterpret_48/1
  in46/1 -> reinterpret_47/1
  in45/1 -> reinterpret_46/1
  in44/1 -> reinterpret_45/1
  in43/1 -> reinterpret_44/1
  in42/1 -> reinterpret_43/1
  in41/1 -> reinterpret_42/1
  in40/1 -> reinterpret_41/1
  in39/1 -> reinterpret_40/1
  in38/1 -> reinterpret_39/1
  in37/1 -> reinterpret_38/1
  in36/1 -> reinterpret_37/1
  in35/1 -> reinterpret_36/1
  in34/1 -> reinterpret_35/1
  in33/1 -> reinterpret_34/1
  in32/1 -> reinterpret_33/1
  in31/1 -> reinterpret_32/1
  in30/1 -> reinterpret_31/1
  in29/1 -> reinterpret_30/1
  in28/1 -> reinterpret_29/1
  in27/1 -> reinterpret_28/1
  in26/1 -> reinterpret_27/1
  in25/1 -> reinterpret_26/1
  in24/1 -> reinterpret_25/1
  in23/1 -> reinterpret_24/1
  in22/1 -> reinterpret_23/1
  in21/1 -> reinterpret_22/1
  in20/1 -> reinterpret_21/1
  in19/1 -> reinterpret_20/1
  in18/1 -> reinterpret_19/1
  in17/1 -> reinterpret_18/1
  in16/1 -> reinterpret_17/1
  in15/1 -> reinterpret_16/1
  in14/1 -> reinterpret_15/1
  in13/1 -> reinterpret_14/1
  in12/1 -> reinterpret_13/1
  in11/1 -> reinterpret_12/1
  in10/1 -> reinterpret_11/1
  in9/1 -> reinterpret_10/1
  in8/1 -> reinterpret_9/1
  in7/1 -> reinterpret_8/1
  in6/1 -> reinterpret_7/1
  in5/1 -> reinterpret_6/1
  in4/1 -> reinterpret_5/1
  in3/1 -> reinterpret_4/1
  in2/1 -> reinterpret_3/1
  in1/1 -> reinterpret_2/1
  in0/1 -> reinterpret_1/1
